simulink model "Second"  (R2016a)
settings: Solver=VariableStepAuto  StartTime=0.0  StopTime=1  MaxStep=1e-6  RelTol=1e-3
libraries: powerlib x30, simulink x6, powerlib_meascontrol x4
settings Model: Creator=Junhong  LastModifiedBy=Junhong

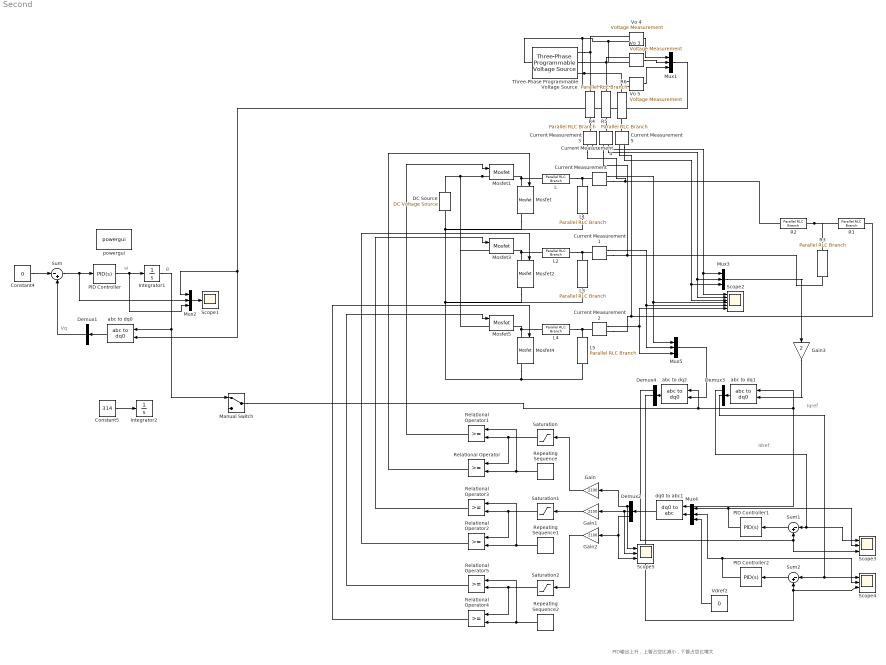
== system Second ==
  note: Idref
  note: Iqref
  note: PID输出上升，上管占空比减小，下管占空比增大
  note: θ
  note: ω
  note: Vq
  Constant4 : Constant  Value=0
  Constant5 : Constant  Value=314
  Current Measurement{,1..5} (6 alike) : powerlib/Measurements/Current Measurement  PhasorSimulation=off  OutputType=Complex  PSBequivalent=0
  DC Source : powerlib/Electrical Sources/DC Voltage Source  Amplitude=40  Measurements=None
  Demux{1..4} (4 alike) : Demux  Outputs=3
  Gain : Gain  Gain=2100
  Gain1 : Gain  Gain=2100
  Gain2 : Gain  Gain=2100
  Gain3 : Gain  Gain=2
  Integrator1 : Integrator
  Integrator2 : Integrator
  L : powerlib/Elements/Parallel RLC Branch  LConnTagsString=a  RConnTagsString=__new0  BranchType=L  Resistance=1  Inductance=500e-6  SetiL0=off  InitialCurrent=0  Capacitance=1e-6  Setx0=off  InitialVoltage=0  Measurements=None
  L1 : powerlib/Elements/Parallel RLC Branch  LConnTagsString=a  RConnTagsString=__new0  BranchType=C  Resistance=0.047  Inductance=1e-3  SetiL0=off  InitialCurrent=0  Capacitance=10e-6  Setx0=off  InitialVoltage=0  Measurements=None
  L2 : powerlib/Elements/Parallel RLC Branch  LConnTagsString=a  RConnTagsString=__new0  BranchType=L  Resistance=1  Inductance=500e-6  SetiL0=off  InitialCurrent=0  Capacitance=1e-6  Setx0=off  InitialVoltage=0  Measurements=None
  L3 : powerlib/Elements/Parallel RLC Branch  LConnTagsString=a  RConnTagsString=__new0  BranchType=C  Resistance=0.047  Inductance=1e-3  SetiL0=off  InitialCurrent=0  Capacitance=10e-6  Setx0=off  InitialVoltage=0  Measurements=None
  L4 : powerlib/Elements/Parallel RLC Branch  LConnTagsString=a  RConnTagsString=__new0  BranchType=L  Resistance=1  Inductance=500e-6  SetiL0=off  InitialCurrent=0  Capacitance=1e-6  Setx0=off  InitialVoltage=0  Measurements=None
  L5 : powerlib/Elements/Parallel RLC Branch  LConnTagsString=a  RConnTagsString=__new0  BranchType=C  Resistance=0.047  Inductance=1e-3  SetiL0=off  InitialCurrent=0  Capacitance=10e-6  Setx0=off  InitialVoltage=0  Measurements=None
  Manual Switch : ManualSwitch
  Mosfet{,1..5} (6 alike) : powerlib/Power Electronics/Mosfet  Ron=0.1  Lon=0  Rd=0.01  Vfd=0  IC=0  Rs=1e5  Cs=inf  Measurements=on
  Mux{1..5} (5 alike) : Mux  Inputs=3
  PID Controller : simulink/Continuous/PID Controller  Controller=PID  TimeDomain=Continuous-time  SampleTime=-1  IntegratorMethod=Forward Euler  FilterMethod=Forward Euler  Form=Parallel  UseFilter=on  ControllerParametersSource=internal  P=100  I=1  D=0  N=1000000  InitialConditionSource=internal  InitialConditionForIntegrator=0  InitialConditionForFilter=0  ExternalReset=none  LimitOutput=off  UpperSaturationLimit=inf  LowerSaturationLimit=-inf  LinearizeAsGain=on  AntiWindupMode=none  Kb=1  TrackingMode=off  Kt=1  PParamMin=[]  PParamMax=[]  IParamMin=[]  IParamMax=[]  DParamMin=[]  DParamMax=[]  NParamMin=[]  NParamMax=[]  KbParamMin=[]  KbParamMax=[]  KtParamMin=[]  KtParamMax=[]  POutMin=[]  POutMax=[]  IOutMin=[]  IOutMax=[]  DOutMin=[]  DOutMax=[]  NOutMin=[]  NOutMax=[]  KbOutMin=[]  KbOutMax=[]  KtOutMin=[]  KtOutMax=[]  IntegratorOutMin=[]  IntegratorOutMax=[]  FilterOutMin=[]  FilterOutMax=[]  SumOutMin=[]  SumOutMax=[]  SumI1OutMin=[]  SumI1OutMax=[]  SumI2OutMin=[]  SumI2OutMax=[]  SumI3OutMin=[]  SumI3OutMax=[]  SumDOutMin=[]  SumDOutMax=[]  SaturationOutMin=[]  SaturationOutMax=[]  IntegratorContinuousStateAttributes=''  IntegratorStateMustResolveToSignalObject=off  IntegratorRTWStateStorageClass=Auto  FilterContinuousStateAttributes=''  FilterStateMustResolveToSignalObject=off  FilterRTWStateStorageClass=Auto  DifferentiatorICPrevScaledInput=0  DifferentiatorOutMin=[]  DifferentiatorOutMax=[]
  PID Controller1 : simulink/Continuous/PID Controller  Controller=PID  TimeDomain=Continuous-time  SampleTime=-1  IntegratorMethod=Forward Euler  FilterMethod=Forward Euler  Form=Parallel  UseFilter=on  ControllerParametersSource=internal  P=0.001  I=0.2  D=0  N=1000000  InitialConditionSource=internal  InitialConditionForIntegrator=0  InitialConditionForFilter=0  ExternalReset=none  LimitOutput=off  UpperSaturationLimit=inf  LowerSaturationLimit=-inf  LinearizeAsGain=on  AntiWindupMode=none  Kb=1  TrackingMode=off  Kt=1  PParamMin=[]  PParamMax=[]  IParamMin=[]  IParamMax=[]  DParamMin=[]  DParamMax=[]  NParamMin=[]  NParamMax=[]  KbParamMin=[]  KbParamMax=[]  KtParamMin=[]  KtParamMax=[]  POutMin=[]  POutMax=[]  IOutMin=[]  IOutMax=[]  DOutMin=[]  DOutMax=[]  NOutMin=[]  NOutMax=[]  KbOutMin=[]  KbOutMax=[]  KtOutMin=[]  KtOutMax=[]  IntegratorOutMin=[]  IntegratorOutMax=[]  FilterOutMin=[]  FilterOutMax=[]  SumOutMin=[]  SumOutMax=[]  SumI1OutMin=[]  SumI1OutMax=[]  SumI2OutMin=[]  SumI2OutMax=[]  SumI3OutMin=[]  SumI3OutMax=[]  SumDOutMin=[]  SumDOutMax=[]  SaturationOutMin=[]  SaturationOutMax=[]  IntegratorContinuousStateAttributes=''  IntegratorStateMustResolveToSignalObject=off  IntegratorRTWStateStorageClass=Auto  FilterContinuousStateAttributes=''  FilterStateMustResolveToSignalObject=off  FilterRTWStateStorageClass=Auto  DifferentiatorICPrevScaledInput=0  DifferentiatorOutMin=[]  DifferentiatorOutMax=[]
  PID Controller2 : simulink/Continuous/PID Controller  Controller=PID  TimeDomain=Continuous-time  SampleTime=-1  IntegratorMethod=Forward Euler  FilterMethod=Forward Euler  Form=Parallel  UseFilter=on  ControllerParametersSource=internal  P=0.001  I=0.2  D=0  N=1000000  InitialConditionSource=internal  InitialConditionForIntegrator=0  InitialConditionForFilter=0  ExternalReset=none  LimitOutput=off  UpperSaturationLimit=inf  LowerSaturationLimit=-inf  LinearizeAsGain=on  AntiWindupMode=none  Kb=1  TrackingMode=off  Kt=1  PParamMin=[]  PParamMax=[]  IParamMin=[]  IParamMax=[]  DParamMin=[]  DParamMax=[]  NParamMin=[]  NParamMax=[]  KbParamMin=[]  KbParamMax=[]  KtParamMin=[]  KtParamMax=[]  POutMin=[]  POutMax=[]  IOutMin=[]  IOutMax=[]  DOutMin=[]  DOutMax=[]  NOutMin=[]  NOutMax=[]  KbOutMin=[]  KbOutMax=[]  KtOutMin=[]  KtOutMax=[]  IntegratorOutMin=[]  IntegratorOutMax=[]  FilterOutMin=[]  FilterOutMax=[]  SumOutMin=[]  SumOutMax=[]  SumI1OutMin=[]  SumI1OutMax=[]  SumI2OutMin=[]  SumI2OutMax=[]  SumI3OutMin=[]  SumI3OutMax=[]  SumDOutMin=[]  SumDOutMax=[]  SaturationOutMin=[]  SaturationOutMax=[]  IntegratorContinuousStateAttributes=''  IntegratorStateMustResolveToSignalObject=off  IntegratorRTWStateStorageClass=Auto  FilterContinuousStateAttributes=''  FilterStateMustResolveToSignalObject=off  FilterRTWStateStorageClass=Auto  DifferentiatorICPrevScaledInput=0  DifferentiatorOutMin=[]  DifferentiatorOutMax=[]
  R1 : powerlib/Elements/Parallel RLC Branch  LConnTagsString=a  RConnTagsString=__new0  BranchType=R  Resistance=8  Inductance=0.00033  SetiL0=off  InitialCurrent=0  Capacitance=1e-6  Setx0=off  InitialVoltage=0  Measurements=None
  R2 : powerlib/Elements/Parallel RLC Branch  LConnTagsString=a  RConnTagsString=__new0  BranchType=R  Resistance=8  Inductance=0.00033  SetiL0=off  InitialCurrent=0  Capacitance=1e-6  Setx0=off  InitialVoltage=0  Measurements=None
  R3 : powerlib/Elements/Parallel RLC Branch  LConnTagsString=a  RConnTagsString=__new0  BranchType=R  Resistance=8  Inductance=0.00033  SetiL0=off  InitialCurrent=0  Capacitance=1e-6  Setx0=off  InitialVoltage=0  Measurements=None
  R4 : powerlib/Elements/Parallel RLC Branch  LConnTagsString=a  RConnTagsString=__new0  BranchType=R  Resistance=0.01  Inductance=0.00033  SetiL0=off  InitialCurrent=0  Capacitance=1e-6  Setx0=off  InitialVoltage=0  Measurements=None
  R5 : powerlib/Elements/Parallel RLC Branch  LConnTagsString=a  RConnTagsString=__new0  BranchType=R  Resistance=0.01  Inductance=0.00033  SetiL0=off  InitialCurrent=0  Capacitance=1e-6  Setx0=off  InitialVoltage=0  Measurements=None
  R6 : powerlib/Elements/Parallel RLC Branch  LConnTagsString=a  RConnTagsString=__new0  BranchType=R  Resistance=0.01  Inductance=0.00033  SetiL0=off  InitialCurrent=0  Capacitance=1e-6  Setx0=off  InitialVoltage=0  Measurements=None
  Relational Operator{,1..5} (6 alike) : RelationalOperator  OutDataTypeStr=boolean
  Repeating Sequence : simulink/Sources/Repeating Sequence  rep_seq_t=[0 2.5e-5]  rep_seq_y=[-1050 1050]
  Repeating Sequence1 : simulink/Sources/Repeating Sequence  rep_seq_t=[0 2.5e-5]  rep_seq_y=[-1050 1050]
  Repeating Sequence2 : simulink/Sources/Repeating Sequence  rep_seq_t=[0 2.5e-5]  rep_seq_y=[-1050 1050]
  Saturation : Saturate  UpperLimit=1050  LowerLimit=-1050
  Saturation1 : Saturate  UpperLimit=1050  LowerLimit=-1050
  Saturation2 : Saturate  UpperLimit=1050  LowerLimit=-1050
  Scope1 : Scope
  Scope2 : Scope  NumInputPorts=6
  Scope3 : Scope  NumInputPorts=3
  Scope4 : Scope  NumInputPorts=3
  Scope5 : Scope  NumInputPorts=3
  Sum : Sum  Inputs=|-+
  Sum1 : Sum  Inputs=|-+
  Sum2 : Sum  Inputs=|-+
  Three-Phase Programmable Voltage Source : powerlib/Electrical Sources/Three-Phase Programmable Voltage Source  PositiveSequence="[19.59  45 50]"  VariationEntity=None  VariationType=Table of time-amplitude pairs  VariationTypeAlt=Step  VariationStep=0.5  VariationRate=10  VariationMagnitude=0.3  VariationFrequency=2  VariationTiming=[1 2]  VariationPhaseA=off  Amplitudes=[1 0.8 1.2 1.0]  TimeValues=[0 0.1 0.15 0.2]  HarmonicGeneration=off  HarmonicA=[3 0.2 -25 0]  HarmonicB=[2 0.15 35 2]  Timing="[0.05  3]"  BusType=swing  Pref=0  Qref=0  Qmin=-inf  Qmax=inf
  Vdref2 : Constant  Value=0
  Vo 3 : powerlib/Measurements/Voltage Measurement  PhasorSimulation=off  OutputType=Complex  PSBequivalent=0
  Vo 4 : powerlib/Measurements/Voltage Measurement  PhasorSimulation=off  OutputType=Complex  PSBequivalent=0
  Vo 5 : powerlib/Measurements/Voltage Measurement  PhasorSimulation=off  OutputType=Complex  PSBequivalent=0
  abc to dq0 : powerlib_meascontrol/Transformations/abc to dq0  Alignment=Aligned with phase A axis
  abc to dq1 : powerlib_meascontrol/Transformations/abc to dq0  Alignment=Aligned with phase A axis
  abc to dq2 : powerlib_meascontrol/Transformations/abc to dq0  Alignment=Aligned with phase A axis
  dq0 to abc1 : powerlib_meascontrol/Transformations/dq0 to abc  Alignment=Aligned with phase A axis
  powergui : powerlib/powergui  Priority=1  SimulationMode=Continuous  SolverType=Tustin/Backward Euler (TBE)  SampleTime=50e-6  frequency=60  SPID=off  DisableSnubberDevices=off  DisableRonSwitches=off  DisableVfSwitches=off  SwTol=0  DisplayEquations=off  Interpol=off  ExternalGateDelay=off  methode=off  Ts=10  FunctionMessages=off  echomessages=off  HookPort=off  EnableUseOfTLC=off  x0status=blocks  frequencyindice=50  Pbase=100e6  ErrMax=1e-4  Iterations=50  UnitsV=kV  UnitsW=MW  buscounter=0  RestoreLinks=warning  ResistiveCurrentMeasurement=off  Frange=[0:2:500]  Ylog=off  Xlog=on  ShowGrid=off  save=off  variable=ZData  structure=0  ZoomFFT=off  StartTime=0.0  cycles=1  DisplayStyle=1  fundamental=60  FreqAxis=off  MaxFrequency=1000  frequencyindicesteady=1  RmsSteady=1  display=off
  wires:
  Saturation/1 -> Relational Operator/1, Relational Operator1/2
  Current Measurement3/1 -> Mux3/1, Scope2/1
  Repeating Sequence/1 -> Relational Operator1/1, Relational Operator/2
  Relational Operator/1 -> Mosfet/1
  Relational Operator1/1 -> Mosfet1/1
  Current Measurement4/1 -> Mux3/2, Scope2/2
  Current Measurement5/1 -> Mux3/3, Scope2/3
  Manual Switch/1 -> abc to dq2/2, abc to dq1/2, dq0 to abc1/2
  Mux3/1 -> Gain3/1
  Saturation1/1 -> Relational Operator2/1, Relational Operator3/2
  Repeating Sequence1/1 -> Relational Operator3/1, Relational Operator2/2
  Relational Operator2/1 -> Mosfet2/1
  Relational Operator3/1 -> Mosfet3/1
  Saturation2/1 -> Relational Operator4/1, Relational Operator5/2
  Repeating Sequence2/1 -> Relational Operator5/1, Relational Operator4/2
  Relational Operator4/1 -> Mosfet4/1
  Relational Operator5/1 -> Mosfet5/1
  dq0 to abc1/1 -> Demux2/1
  abc to dq1/1 -> Demux3/1
  Mux4/1 -> dq0 to abc1/1
  PID Controller2/1 -> Mux4/2, Scope4/2
  Sum1/1 -> PID Controller1/1
  Sum2/1 -> PID Controller2/1
  Demux3/1 -> Scope3/1, Sum1/1
  Demux3/2 -> Sum2/1, Scope4/1
  Gain/1 -> Saturation/1
  Demux2/2 -> Scope5/2, Gain1/1
  Gain1/1 -> Saturation1/1
  Demux2/3 -> Scope5/3, Gain2/1
  Gain2/1 -> Saturation2/1
  Demux2/1 -> Scope5/1, Gain/1
  Vdref2/1 -> Mux4/3
  PID Controller1/1 -> Mux4/1, Scope3/2
  Constant4/1 -> Sum/1
  abc to dq0/1 -> Demux1/1
  Sum/1 -> Mux2/2, PID Controller/1
  PID Controller/1 -> Mux2/3, Integrator1/1
  Mux2/1 -> Scope1/1
  Demux1/2 -> Sum/2
  Vo 4/1 -> Mux1/1
  Vo 3/1 -> Mux1/2
  Vo 5/1 -> Mux1/3
  Mux1/1 -> abc to dq0/1, Mux2/1
  Gain3/1 -> abc to dq1/1
  Mux5/1 -> abc to dq2/1
  Current Measurement/1 -> Scope2/4, Mux5/1
  Current Measurement1/1 -> Scope2/5, Mux5/2
  Current Measurement2/1 -> Scope2/6, Mux5/3
  abc to dq2/1 -> Demux4/1
  Demux4/1 -> Scope3/3, Sum1/2
  Demux4/2 -> Scope4/3, Sum2/2
  Constant5/1 -> Integrator2/1
  Integrator1/1 -> abc to dq0/2, Manual Switch/1
  connections:
  L/RConn1 -- Current Measurement/LConn1 -- L1/LConn1
  Mosfet4/RConn1 -- L5/RConn1 -- DC Source/LConn1 -- Mosfet/RConn1 -- L1/RConn1 -- Mosfet2/RConn1 -- L3/RConn1
  L/LConn1 -- Mosfet/LConn1 -- Mosfet1/RConn1
  Mosfet1/LConn1 -- DC Source/RConn1 -- Mosfet3/LConn1 -- Mosfet5/LConn1
  L2/LConn1 -- Mosfet2/LConn1 -- Mosfet3/RConn1
  L4/LConn1 -- Mosfet4/LConn1 -- Mosfet5/RConn1
  L2/RConn1 -- Current Measurement1/LConn1 -- L3/LConn1
  L4/RConn1 -- Current Measurement2/LConn1 -- L5/LConn1
  R2/RConn1 -- R1/LConn1 -- R3/LConn1
  Vo 4/LConn2 -- Three-Phase Programmable Voltage Source/LConn1 -- Vo 5/LConn2 -- Vo 3/LConn2
  R2/LConn1 -- Current Measurement3/RConn1 -- Current Measurement/RConn1
  Current Measurement1/RConn1 -- Current Measurement4/RConn1 -- R3/RConn1
  Current Measurement2/RConn1 -- R1/RConn1 -- Current Measurement5/RConn1
  Three-Phase Programmable Voltage Source/RConn1 -- Vo 4/LConn1 -- R4/LConn1
  R5/RConn1 -- Current Measurement4/LConn1
  Three-Phase Programmable Voltage Source/RConn3 -- R6/LConn1 -- Vo 5/LConn1
  R4/RConn1 -- Current Measurement3/LConn1
  Vo 3/LConn1 -- R5/LConn1 -- Three-Phase Programmable Voltage Source/RConn2
  Current Measurement5/LConn1 -- R6/RConn1
